simulink model "sldemo_mdlref_depgraph"  (Simulink 7.6)
settings: Solver=ode3  SolverMode=SingleTasking  StartTime=0.0  StopTime=2*24*60*60  FixedStep=60  RelTol=1e-3  AbsTol=1e-6
settings Model: Creator=The MathWorks Inc.  ExtModeTrigMode=oneshot  ExtModeArmWhenConnect=off  ExtModeAutoUpdateStatusClock=off
settings DataIOCC: ExternalInput=[]  InitialState=[]  LimitDataPoints=off  SaveOutput=off  SaveTime=off
settings OptimizationCC: BlockReduction=off  BooleanDataType=off  InlineParams=on  InlineInvariantSignals=on  InitFltsAndDblsToZero=on
settings DebuggingCC: SaveWithParameterizedLinksMsg=none  CheckExecutionContextPreStartOutputMsg=on  CheckExecutionContextRuntimeOutputMsg=on  SolverPrmCheckMsg=none  DiscreteInheritContinuousMsg=none  MultiTaskDSMMsg=warning  MultiTaskCondExecSysMsg=none  SigSpecEnsureSampleTimeMsg=none  IntegerOverflowMsg=none
settings ModelReferenceCC: UpdateModelReferenceTargets=IfOutOfDate
settings RTWCC: IncludeERTFirstTime=on
settings CodeAppCC: MaxIdLength=100
settings GRTTargetCC: TargetFcnLib=ansi_tfl_tmw.mat

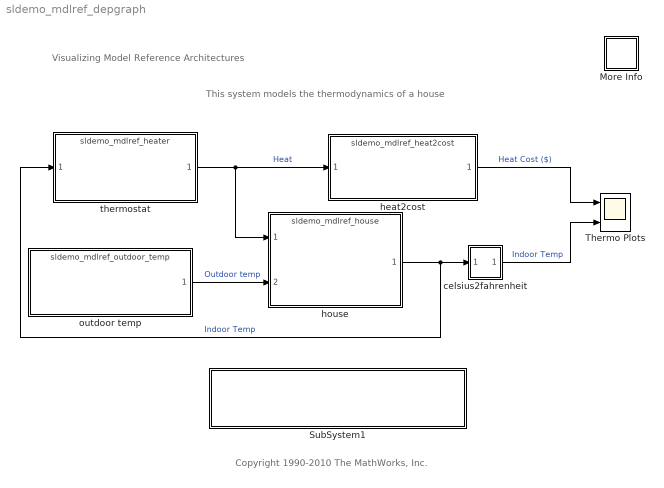
== system sldemo_mdlref_depgraph ==
  note: Visualizing Model Reference Architectures
  note: This system models the thermodynamics of a house
  note: Copyright 1990-2010 The MathWorks, Inc.
  More Info : Subsystem
      settings: OpenFcn=showdemo(bdroot(gcb))
      mask Display: disp('?')
  SubSystem1 : Subsystem
      settings: OpenFcn=|
      | mdlName= get_param(bdroot(gcbh),'name');
      | view_mdlrefs(mdlName);
      mask Display: disp('Double click here to view \n Model Reference dependency graph');
  Thermo Plots : Scope  NumInputPorts=2
      settings: TickLabels=on  TimeRange=200000  YMin=0~60  YMax=40~80
  celsius2fahrenheit : Subsystem
      mask Type: CelsiusToFahrenheit
      mask Description:
      | Conversion from degrees Celsius to degrees Fahrenheit.
      | 
      | F=9/5*C+32
      mask Help: This block converts from degrees Celsius to degrees Fahrenheit.
      mask Display: disp('C2F')
  heat2cost : ModelReference  ModelNameDialog=sldemo_mdlref_heat2cost  SimulationMode=Accelerator  ModelReferenceVersion=1.13  CopyOfModelName=sldemo_mdlref_heat2cost
  house : ModelReference  ModelNameDialog=sldemo_mdlref_house  SimulationMode=Accelerator  ModelReferenceVersion=1.15  CopyOfModelName=sldemo_mdlref_house
  outdoor temp : ModelReference  ModelNameDialog=sldemo_mdlref_outdoor_temp  SimulationMode=Accelerator  ModelReferenceVersion=1.18  CopyOfModelName=sldemo_mdlref_outdoor_temp
  thermostat : ModelReference  ModelNameDialog=sldemo_mdlref_heater  SimulationMode=Normal  ModelReferenceVersion=1.25  CopyOfModelName=sldemo_mdlref_heater
  wires:
  thermostat/1 -> house/1, heat2cost/1  "Heat"
  house/1 -> celsius2fahrenheit/1(Celsius in), thermostat/1  "Indoor Temp"
  outdoor temp/1 -> house/2  "Outdoor temp"
  heat2cost/1 -> Thermo Plots/1  "Heat Cost ($)"
  celsius2fahrenheit/1(Fahrenheit out) -> Thermo Plots/2  "Indoor Temp"

== system sldemo_mdlref_depgraph/More Info ==
  note: Bus Block Demonstration
  note: This demonstration shows how signals may be grouped and ungrouped while
      | retaining their names.  In this demonstration, 5 signals are created and labelled
      | appropriately.  These signals are then mux'd together to create a bus of signals.
      | This bus of signals is then fed into the Bus Selector block.  Inside of the Bus
      | Selector block, the Pulse and Chirp signals are chosen to be output from the
      | original signal bus.
      |
      | It is possible to place a nest signal buses and then still retrieve the original signal
      | with its label.

== system sldemo_mdlref_depgraph/SubSystem1 ==

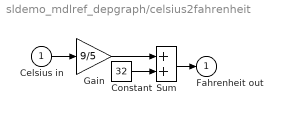
== system sldemo_mdlref_depgraph/celsius2fahrenheit ==
  Celsius in : Inport
  Constant : Constant  Value=32  OutDataTypeStr=Inherit: Inherit via back propagation
  Gain : Gain  Gain=9/5  SaturateOnIntegerOverflow=on  OutDataTypeStr=Inherit: Same as input  ParamDataTypeStr=Inherit: Same as input
  Sum : Sum  SaturateOnIntegerOverflow=on  InputSameDT=on  OutDataTypeStr=Inherit: Same as first input
  Fahrenheit out : Outport  InitialOutput=0
  wires:
  Celsius in/1 -> Gain/1
  Gain/1 -> Sum/1
  Sum/1 -> Fahrenheit out/1
  Constant/1 -> Sum/2
